simulink model "eps_simulation"  (R2014a)
settings: Solver=ode45  StartTime=0.0  StopTime=10  RelTol=1e-3
values from neighbouring files (symbols this model uses):
  Cc = 0.05    [para_init.m]
  Cm = 6.9e-4    (= 0.00069)    [para_init.m]
  Cw = 25    [para_init.m]
  D = 0.01    [para_init.m]
  Fc = 0.6    [para_init.m]
  Fm = 0.07    [para_init.m]
  Fw = 8    [para_init.m]
  g = 9.8    [para_init.m]
  I = 1500    [para_init.m]
  Ic = 2e-4    (= 0.0002)    [para_init.m]
  Ih = 0.03    [para_init.m]
  Im = 3e-4    (= 0.0003)    [para_init.m]
  Iw = 1.3    [para_init.m]
  Kc = 1000    [para_init.m]
  Kf = 34000    [para_init.m]
  Kg = 20000    [para_init.m]
  Kr = 34000    [para_init.m]
  Kts = 120    [para_init.m]
  Lf = 0.86    [para_init.m]
  Lr = 1.5    [para_init.m]
  M = 950    [para_init.m]
  Ng = 16    [para_init.m]
  Nm = 17    [para_init.m]
  sigma = (11+5/6)*pi/180    (= 0.206530628153)    [para_init.m]
  V = 20/3.6    (= 5.55555555556)    [para_init.m]
  Xi = 0.05    [para_init.m]
libraries: simulink x2
settings Model: Creator=Charlie Ren  LastModifiedBy=Charlie Ren

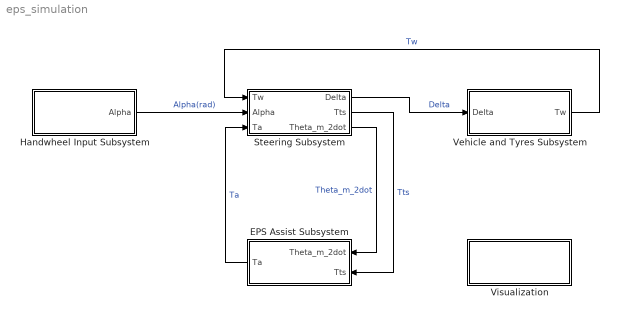
== system eps_simulation ==
  EPS Assist Subsystem : Subsystem
  Handwheel Input Subsystem : Subsystem
  Steering Subsystem : Subsystem
  Vehicle and Tyres Subsystem : Subsystem
  Visualization : Subsystem
  wires:
  Handwheel Input Subsystem/1(Alpha) -> Steering Subsystem/2(Alpha)  "Alpha(rad)"
  Steering Subsystem/1(Delta) -> Vehicle and Tyres Subsystem/1(Delta)  "Delta"
  Vehicle and Tyres Subsystem/1(Tw) -> Steering Subsystem/1(Tw)  "Tw"
  EPS Assist Subsystem/1(Ta) -> Steering Subsystem/3(Ta)  "Ta"
  Steering Subsystem/2(Tts) -> EPS Assist Subsystem/2(Tts)  "Tts"
  Steering Subsystem/3(Theta_m_2dot) -> EPS Assist Subsystem/1(Theta_m_2dot)  "Theta_m_2dot"

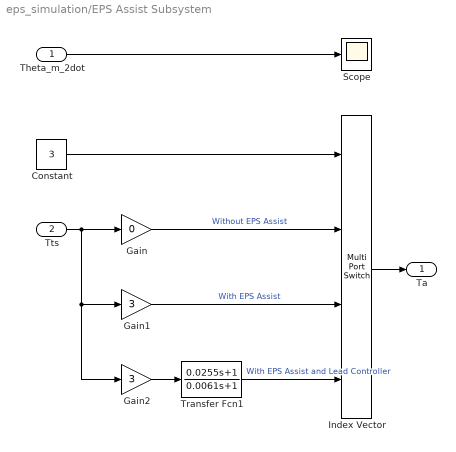
== system eps_simulation/EPS Assist Subsystem ==
  Theta_m_2dot : Inport
  Tts : Inport  Port=2
  Constant : Constant  Value=3
  Gain : Gain  Gain=0
  Gain1 : Gain  Gain=3
  Gain2 : Gain  Gain=3
  Index Vector : MultiPortSwitch
  Scope : Scope
  Transfer Fcn1 : TransferFcn  Numerator=[0.0255 1]  Denominator=[0.0061 1]
  Ta : Outport
  wires:
  Theta_m_2dot/1 -> Scope/1
  Constant/1 -> Index Vector/1
  Tts/1 -> Gain/1, Gain1/1, Gain2/1
  Gain/1 -> Index Vector/2  "Without EPS Assist"
  Gain1/1 -> Index Vector/3  "With EPS Assist"
  Index Vector/1 -> Ta/1
  Gain2/1 -> Transfer Fcn1/1
  Transfer Fcn1/1 -> Index Vector/4  "With EPS Assist and Lead Controller"

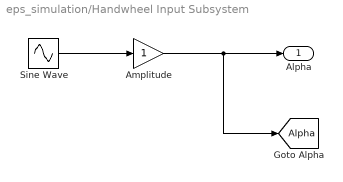
== system eps_simulation/Handwheel Input Subsystem ==
  Amplitude : Gain
  Sine Wave : Sin  SampleTime=0
  Alpha : Outport
  tag scope: Alpha=global
  wires:
  Sine Wave/1 -> Amplitude/1
  Amplitude/1 -> [Alpha], Alpha/1

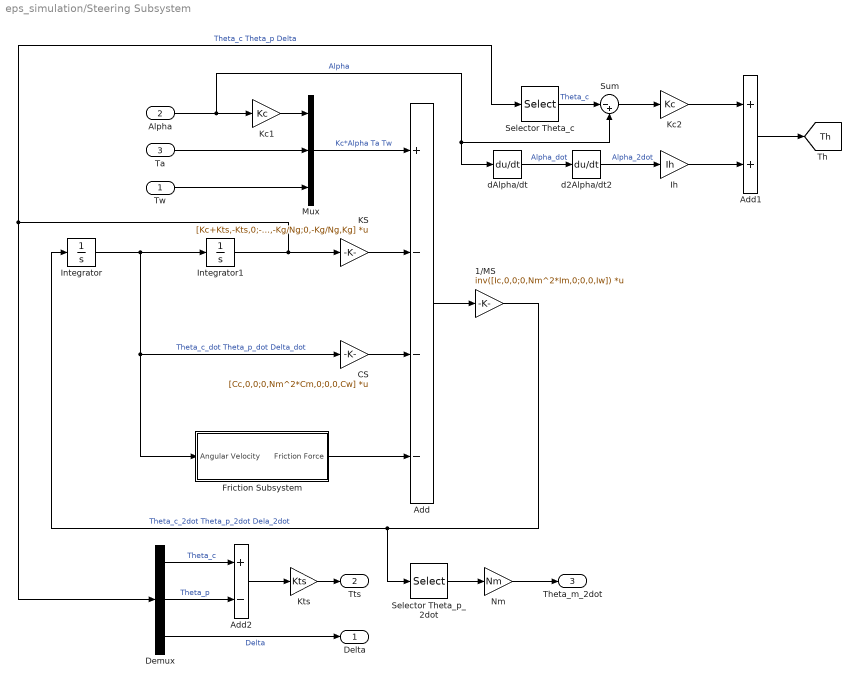
== system eps_simulation/Steering Subsystem ==
  Tw : Inport
  Alpha : Inport  Port=2
  Ta : Inport  Port=3
  1/MS : Gain  Gain=inv([Ic,0,0;0,Nm^2*Im,0;0,0,Iw])  Multiplication=Matrix(K*u)
  Add : Sum  Inputs=+---
  Add1 : Sum
  Add2 : Sum  Inputs=+-
  CS : Gain  Gain=[Cc,0,0;0,Nm^2*Cm,0;0,0,Cw]  Multiplication=Matrix(K*u)
  Demux : Demux  Outputs=3
  Friction Subsystem : Subsystem
  Ih : Gain  Gain=Ih
  Integrator : Integrator
  Integrator1 : Integrator
  KS : Gain  Gain=[Kc+Kts,-Kts,0;-Kts,Kts+Kg/Ng^2,-Kg/Ng;0,-Kg/Ng,Kg]  Multiplication=Matrix(K*u)
  Kc1 : Gain  Gain=Kc
  Kc2 : Gain  Gain=Kc
  Kts : Gain  Gain=Kts
  Mux : Mux  Inputs=3
  Nm : Gain  Gain=Nm
  Selector Theta_p_2dot : Selector  InputPortWidth=3  Indices=[2]
  Selector Theta_c : Selector  InputPortWidth=3  Indices=[1]
  Sum : Sum  Inputs=|-+
  d2Alpha/dt2 : Derivative
  dAlpha/dt : Derivative
  Delta : Outport
  Tts : Outport  Port=2
  Theta_m_2dot : Outport  Port=3
  tag scope: Th=global
  wires:
  Kc1/1 -> Mux/1
  Mux/1 -> Add/1  "Kc*Alpha Ta Tw"
  dAlpha/dt/1 -> d2Alpha/dt2/1  "Alpha_dot"
  d2Alpha/dt2/1 -> Ih/1  "Alpha_2dot"
  Selector Theta_c/1 -> Sum/1  "Theta_c"
  Sum/1 -> Kc2/1
  Kc2/1 -> Add1/1
  Ih/1 -> Add1/2
  KS/1 -> Add/2
  CS/1 -> Add/3
  Integrator/1 -> CS/1, Friction Subsystem/1(Angular Velocity), Integrator1/1  "Theta_c_dot Theta_p_dot Delta_dot"
  Friction Subsystem/1(Friction Force) -> Add/4
  Demux/2 -> Add2/2  "Theta_p"
  Demux/1 -> Add2/1  "Theta_c"
  Add2/1 -> Kts/1
  Demux/3 -> Delta/1  "Delta"
  Kts/1 -> Tts/1
  Add/1 -> 1/MS/1
  1/MS/1 -> Selector Theta_p_2dot/1, Integrator/1  "Theta_c_2dot Theta_p_2dot Dela_2dot"
  Selector Theta_p_2dot/1 -> Nm/1
  Nm/1 -> Theta_m_2dot/1
  Integrator1/1 -> Selector Theta_c/1, Demux/1, KS/1  "Theta_c Theta_p Delta"
  Ta/1 -> Mux/2
  Tw/1 -> Mux/3
  Alpha/1 -> Sum/2, dAlpha/dt/1, Kc1/1  "Alpha"
  Add1/1 -> [Th]

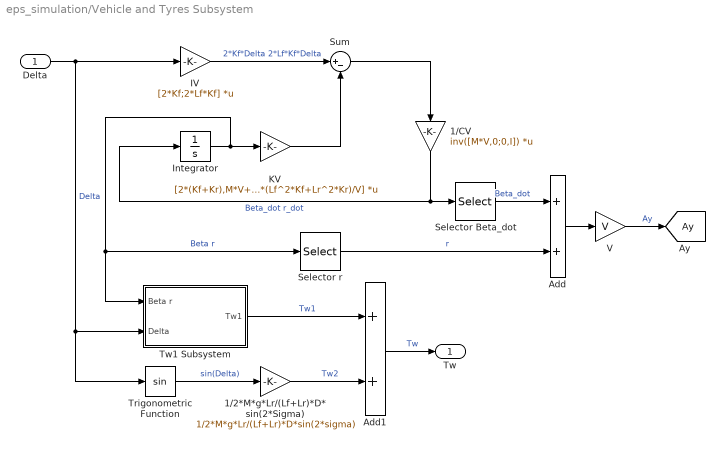
== system eps_simulation/Vehicle and Tyres Subsystem ==
  Delta : Inport
  1/2*M*g*Lr/(Lf+Lr)*D*sin(2*Sigma) : Gain  Gain=1/2*M*g*Lr/(Lf+Lr)*D*sin(2*sigma)
  1/CV : Gain  Gain=inv([M*V,0;0,I])  Multiplication=Matrix(K*u)
  Add : Sum
  Add1 : Sum
  IV : Gain  Gain=[2*Kf;2*Lf*Kf]  Multiplication=Matrix(K*u)
  Integrator : Integrator
  KV : Gain  Gain=[2*(Kf+Kr),M*V+2*(Lf*Kf-Lr*Kr)/V;2*(Lf*Kf-Lr*Kr),2*(Lf^2*Kf+Lr^2*Kr)/V]  Multiplication=Matrix(K*u)
  Selector Beta_dot : Selector  InputPortWidth=2  Indices=[1]
  Selector r : Selector  InputPortWidth=2  Indices=[2]
  Sum : Sum  Inputs=|+-
  Trigonometric Function : Trigonometry
  Tw1 Subsystem : Subsystem
  V : Gain  Gain=V
  Tw : Outport
  tag scope: Ay=global
  wires:
  IV/1 -> Sum/1  "2*Kf*Delta 2*Lf*Kf*Delta"
  Sum/1 -> 1/CV/1
  KV/1 -> Sum/2
  1/CV/1 -> Integrator/1, Selector Beta_dot/1  "Beta_dot r_dot"
  Selector Beta_dot/1 -> Add/1  "Beta_dot"
  Add/1 -> V/1
  Selector r/1 -> Add/2  "r"
  Integrator/1 -> Tw1 Subsystem/1(Beta r), Selector r/1, KV/1  "Beta r"
  Delta/1 -> Trigonometric Function/1, Tw1 Subsystem/2(Delta), IV/1  "Delta"
  Trigonometric Function/1 -> 1/2*M*g*Lr/(Lf+Lr)*D*sin(2*Sigma)/1  "sin(Delta)"
  Tw1 Subsystem/1(Tw1) -> Add1/1  "Tw1"
  1/2*M*g*Lr/(Lf+Lr)*D*sin(2*Sigma)/1 -> Add1/2  "Tw2"
  Add1/1 -> Tw/1  "Tw"
  V/1 -> [Ay]  "Ay"

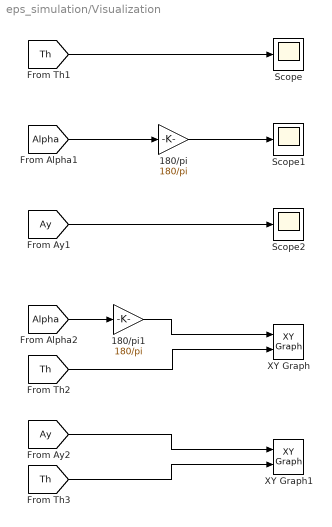
== system eps_simulation/Visualization ==
  180/pi : Gain  Gain=180/pi
  180/pi1 : Gain  Gain=180/pi
  Scope : Scope
  Scope1 : Scope
      settings: SaveName=ScopeData2
  Scope2 : Scope
      settings: SaveName=ScopeData3
  XY Graph : simulink/Sinks/XY Graph  xmin=-1  xmax=1  ymin=-1  ymax=1  st=-1
  XY Graph1 : simulink/Sinks/XY Graph  xmin=-1  xmax=1  ymin=-1  ymax=1  st=-1
  wires:
  [Th] -> Scope/1
  [Ay] -> Scope2/1
  [Alpha] -> 180/pi1/1
  [Th] -> XY Graph/2
  [Ay] -> XY Graph1/1
  [Th] -> XY Graph1/2
  [Alpha] -> 180/pi/1
  180/pi/1 -> Scope1/1
  180/pi1/1 -> XY Graph/1

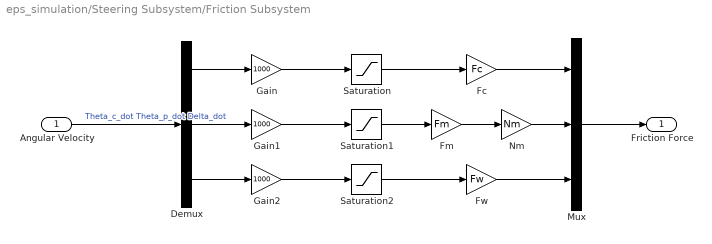
== system eps_simulation/Steering Subsystem/Friction Subsystem ==
  Angular Velocity : Inport
  Demux : Demux  Outputs=3
  Fc : Gain  Gain=Fc
  Fm : Gain  Gain=Fm
  Fw : Gain  Gain=Fw
  Gain : Gain  Gain=1000
  Gain1 : Gain  Gain=1000
  Gain2 : Gain  Gain=1000
  Mux : Mux  Inputs=3
  Nm : Gain  Gain=Nm
  Saturation : Saturate  UpperLimit=1  LowerLimit=-1
  Saturation1 : Saturate  UpperLimit=1  LowerLimit=-1
  Saturation2 : Saturate  UpperLimit=1  LowerLimit=-1
  Friction Force : Outport
  wires:
  Angular Velocity/1 -> Demux/1  "Theta_c_dot Theta_p_dot Delta_dot"
  Demux/1 -> Gain/1
  Demux/2 -> Gain1/1
  Demux/3 -> Gain2/1
  Gain/1 -> Saturation/1
  Gain1/1 -> Saturation1/1
  Gain2/1 -> Saturation2/1
  Saturation/1 -> Fc/1
  Saturation1/1 -> Fm/1
  Saturation2/1 -> Fw/1
  Fm/1 -> Nm/1
  Nm/1 -> Mux/2
  Fc/1 -> Mux/1
  Fw/1 -> Mux/3
  Mux/1 -> Friction Force/1

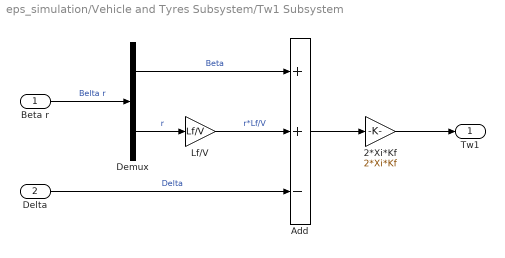
== system eps_simulation/Vehicle and Tyres Subsystem/Tw1 Subsystem ==
  Beta r : Inport
  Delta : Inport  Port=2
  2*Xi*Kf : Gain  Gain=2*Xi*Kf
  Add : Sum  Inputs=++-
  Demux : Demux  Outputs=2
  Lf/V : Gain  Gain=Lf/V
  Tw1 : Outport
  wires:
  Beta r/1 -> Demux/1  "Belta r"
  Demux/1 -> Add/1  "Beta"
  Demux/2 -> Lf/V/1  "r"
  Lf/V/1 -> Add/2  "r*Lf/V"
  Delta/1 -> Add/3  "Delta"
  Add/1 -> 2*Xi*Kf/1
  2*Xi*Kf/1 -> Tw1/1
